simulink model "SyntheticDataSimulinkExample"  (R2017b)
settings: Solver=FixedStepDiscrete  StartTime=0.0  StopTime=14.34  FixedStep=0.1  RelTol=1e-3
undefined symbols (not defined in the file or in its folder): driving
libraries: drivinglib x12, drivingmisc x1
settings Model: Creator=The MathWorks, Inc.  LastModifiedBy=The MathWorks, Inc.
settings CodeAppCC: StateflowObjectComments=on

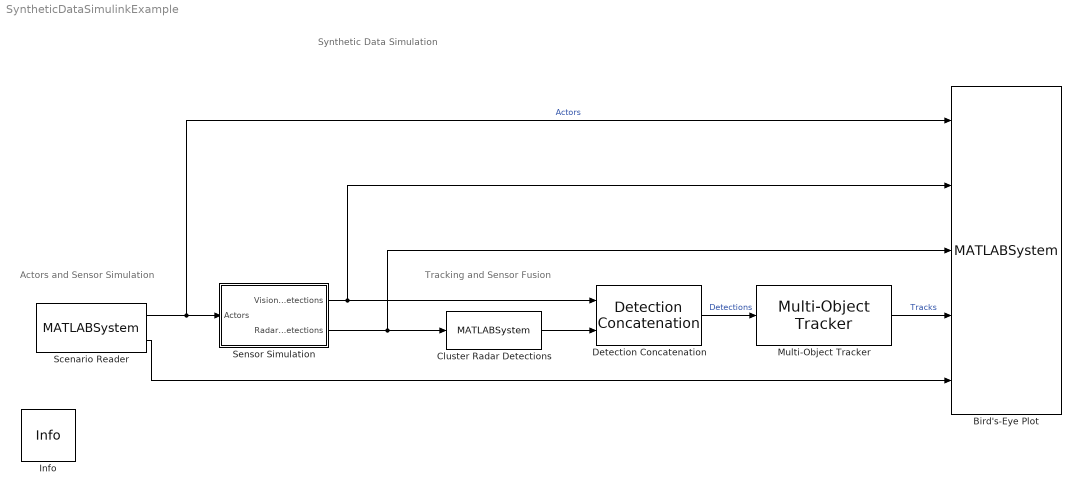
== system SyntheticDataSimulinkExample ==
  note: Tracking and Sensor Fusion
  note: Actors and Sensor Simulation
  note: Synthetic Data Simulation
  Bird's-Eye Plot : MATLABSystem  System=helperBirdsEyePlot  XLim=[ -60, 60 ]  YLim=[ -50, 50 ]  HasActors=on  HasVision=on  HasRadar=on  HasTracks=on  TrackPositionSelector=[ 1, 0, 0, 0, 0, 0; 0, 0, 1, 0, 0, 0 ]  TrackVelocitySelector=[ 0, 1, 0, 0, 0, 0; 0, 0, 0, 1, 0, 0 ]  HasMIO=off  HasRoads=on
      settings: ModelCloseFcn=helperCloseAll(gcb)
      mask Type: helperBirdsEyePlot
      mask Display:
      | disp(['Bird''s-Eye' char(10) 'Plot']);
      | port_label('input',1,'Actors');
      | port_label('input',2,'Vision');
      | port_label('input',3,'Radar');
      | port_label('input',4,'Tracks');
      | port_label('input',5,'Roads');
  Cluster Radar Detections : MATLABSystem  System=helperClusterDetections  ClusterSize=5  BusNameSource=Auto  SimulateUsing=Interpreted execution
      mask Type: helperClusterDetections
      mask Display:
      | disp(['Detection' char(10) 'Clustering']);
      | port_label('input',1,'In');
      | port_label('output',1,'Out');
  Detection Concatenation : drivinglib/Detection Concatenation  NumInputs=2  BusNameSource=Auto  BusName=BusDetectionConcatenation1  SimulateUsing=Interpreted execution
      settings: SourceProductName=Automated Driving System Toolbox
  Info : drivingmisc/Info  SystemSampleTime=-1
      settings: SourceProductName=Computer Vision System Toolbox  SourceProductBaseCode=VP
  Multi-Object Tracker : drivinglib/Multi-Object Tracker  FilterInitializationFcn=helperInitSimulinkDemoFilter  AssignmentThreshold=50  ConfirmationParameters=[ 2, 3 ]  NumCoastingUpdates=5  MaxNumTracks=20  MaxNumSensors=8  TimeInputSource=Auto  BusNameSource=Auto  BusName=BusMultiObjectTracker1  HasCostMatrixInput=off  TentativeTracksOutputPort=off  AllTracksOutputPort=off  SimulateUsing=Interpreted execution
      settings: SourceProductName=Automated Driving System Toolbox
  Scenario Reader : MATLABSystem  System=helperScenarioReader  ScenarioFileName=openLoopSimulinkScenario  EgoActorSource=Auto  EgoActorID=1  RoadBoundaries=on  BusNameSource=Auto  SimulateUsing=Interpreted execution
      mask Type: helperScenarioReader
      mask Display:
      | disp(['Scenario' char(10) 'Reader']);
      | port_label('output',1,'Actors');
      | port_label('output',2,'Roads');
  Sensor Simulation : Subsystem
  wires:
  Detection Concatenation/1 -> Multi-Object Tracker/1  "Detections"
  Scenario Reader/1 -> Bird's-Eye Plot/1, Sensor Simulation/1(Actors)  "Actors"
  Sensor Simulation/1(Vision Detections) -> Detection Concatenation/1, Bird's-Eye Plot/2
  Sensor Simulation/2(Radar Detections) -> Bird's-Eye Plot/3, Cluster Radar Detections/1
  Cluster Radar Detections/1 -> Detection Concatenation/2
  Scenario Reader/2 -> Bird's-Eye Plot/5
  Multi-Object Tracker/1 -> Bird's-Eye Plot/4  "Tracks"

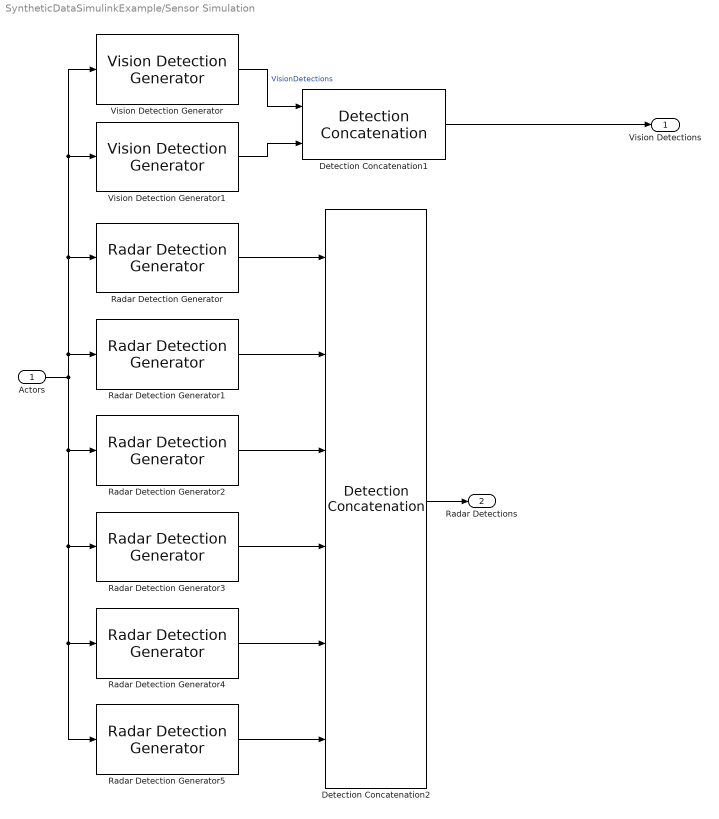
== system SyntheticDataSimulinkExample/Sensor Simulation ==
  Actors : Inport
  Detection Concatenation1 : drivinglib/Detection Concatenation  NumInputs=2  BusNameSource=Auto  BusName=BusDetectionConcatenation3  SimulateUsing=Interpreted execution
      settings: SourceProductName=Automated Driving System Toolbox
  Detection Concatenation2 : drivinglib/Detection Concatenation  NumInputs=6  BusNameSource=Auto  BusName=BusDetectionConcatenation2  SimulateUsing=Interpreted execution
      settings: SourceProductName=Automated Driving System Toolbox
  Radar Detection Generator : drivinglib/Radar Detection Generator  SensorIndex=3  UpdateInterval=0.1  SensorLocation=[ 3.7, 0 ]  Height=0.2  Yaw=0  Pitch=0  Roll=0  BusNameSource=Auto  BusName=BusRadarDetectionGenerator1  MaxNumDetectionsSource=Property  MaxNumDetections=50  DetectionCoordinates=Ego Cartesian  SimulateUsing=Interpreted execution  AzimuthResolution=4  ElevationResolution=10  RangeResolution=2.5  RangeRateResolution=0.5  AzimuthBiasFraction=0.1  ElevationBiasFraction=0.1  RangeBiasFraction=0.05  RangeRateBiasFraction=0.05  FieldOfView=[ 20, 5 ]  MaxRange=174  RangeRateLimits=[ -100, 100 ]  DetectionProbability=0.9  FalseAlarmRate=1e-6  ReferenceRange=100  ReferenceRCS=0  HasElevation=off  HasRangeRate=on  HasNoise=on  HasFalseAlarms=on  InitialSeedSource=Repeatable  InitialSeed=0  UsedSeed=driving.internal.SimulinkUtilities.seedManager(gcb)  ActorProfilesSource=Parameters  ActorProfilesParameters=driving.internal.ActorProfilesRadarParameters  ActorProfilesExpression=struct( 'ClassID', 0, 'Length', 4.7, 'Width', 1.8, 'Height', 1.4, 'OriginOffset', [ -1.35, 0, 0 ], 'RCSPattern', [ 10, 10; 10, 10 ], 'RCSAzimuthAngles', [ -180, 180 ], 'RCSElevationAngles', [ -90, 90 ] )
      settings: SourceProductName=Automated Driving System Toolbox
  Radar Detection Generator1 : drivinglib/Radar Detection Generator  SensorIndex=4  UpdateInterval=0.1  SensorLocation=[-1, 0 ]  Height=0.2  Yaw=180  Pitch=0  Roll=0  BusNameSource=Auto  BusName=BusRadarDetectionGenerator1  MaxNumDetectionsSource=Property  MaxNumDetections=50  DetectionCoordinates=Ego Cartesian  SimulateUsing=Interpreted execution  AzimuthResolution=4  ElevationResolution=10  RangeResolution=2.5  RangeRateResolution=0.5  AzimuthBiasFraction=0.1  ElevationBiasFraction=0.1  RangeBiasFraction=0.05  RangeRateBiasFraction=0.05  FieldOfView=[ 20, 5 ]  MaxRange=174  RangeRateLimits=[ -100, 100 ]  DetectionProbability=0.9  FalseAlarmRate=1e-6  ReferenceRange=100  ReferenceRCS=0  HasElevation=off  HasRangeRate=on  HasNoise=on  HasFalseAlarms=on  InitialSeedSource=Repeatable  InitialSeed=0  UsedSeed=driving.internal.SimulinkUtilities.seedManager(gcb)  ActorProfilesSource=Parameters  ActorProfilesParameters=driving.internal.ActorProfilesRadarParameters  ActorProfilesExpression=struct( 'ClassID', 0, 'Length', 4.7, 'Width', 1.8, 'Height', 1.4, 'OriginOffset', [ -1.35, 0, 0 ], 'RCSPattern', [ 10, 10; 10, 10 ], 'RCSAzimuthAngles', [ -180, 180 ], 'RCSElevationAngles', [ -90, 90 ] )
      settings: SourceProductName=Automated Driving System Toolbox
  Radar Detection Generator2 : drivinglib/Radar Detection Generator  SensorIndex=5  UpdateInterval=0.1  SensorLocation=[0, 0.90 ]  Height=0.2  Yaw=120  Pitch=0  Roll=0  BusNameSource=Auto  BusName=BusRadarDetectionGenerator1  MaxNumDetectionsSource=Property  MaxNumDetections=50  DetectionCoordinates=Ego Cartesian  SimulateUsing=Interpreted execution  AzimuthResolution=4  ElevationResolution=10  RangeResolution=2.5  RangeRateResolution=0.5  AzimuthBiasFraction=0.1  ElevationBiasFraction=0.1  RangeBiasFraction=0.05  RangeRateBiasFraction=0.05  FieldOfView=[ 90, 5 ]  MaxRange=30  RangeRateLimits=[ -100, 100 ]  DetectionProbability=0.9  FalseAlarmRate=1e-6  ReferenceRange=100  ReferenceRCS=0  HasElevation=off  HasRangeRate=on  HasNoise=on  HasFalseAlarms=on  InitialSeedSource=Repeatable  InitialSeed=0  UsedSeed=driving.internal.SimulinkUtilities.seedManager(gcb)  ActorProfilesSource=Parameters  ActorProfilesParameters=driving.internal.ActorProfilesRadarParameters  ActorProfilesExpression=struct( 'ClassID', 0, 'Length', 4.7, 'Width', 1.8, 'Height', 1.4, 'OriginOffset', [ -1.35, 0, 0 ], 'RCSPattern', [ 10, 10; 10, 10 ], 'RCSAzimuthAngles', [ -180, 180 ], 'RCSElevationAngles', [ -90, 90 ] )
      settings: SourceProductName=Automated Driving System Toolbox
  Radar Detection Generator3 : drivinglib/Radar Detection Generator  SensorIndex=6  UpdateInterval=0.1  SensorLocation=[ 0, -0.90 ]  Height=0.2  Yaw=-120  Pitch=0  Roll=0  BusNameSource=Auto  BusName=BusRadarDetectionGenerator1  MaxNumDetectionsSource=Property  MaxNumDetections=50  DetectionCoordinates=Ego Cartesian  SimulateUsing=Interpreted execution  AzimuthResolution=4  ElevationResolution=10  RangeResolution=2.5  RangeRateResolution=0.5  AzimuthBiasFraction=0.1  ElevationBiasFraction=0.1  RangeBiasFraction=0.05  RangeRateBiasFraction=0.05  FieldOfView=[ 90, 5 ]  MaxRange=30  RangeRateLimits=[ -100, 100 ]  DetectionProbability=0.9  FalseAlarmRate=1e-6  ReferenceRange=100  ReferenceRCS=0  HasElevation=off  HasRangeRate=on  HasNoise=on  HasFalseAlarms=on  InitialSeedSource=Repeatable  InitialSeed=0  UsedSeed=driving.internal.SimulinkUtilities.seedManager(gcb)  ActorProfilesSource=Parameters  ActorProfilesParameters=driving.internal.ActorProfilesRadarParameters  ActorProfilesExpression=struct( 'ClassID', 0, 'Length', 4.7, 'Width', 1.8, 'Height', 1.4, 'OriginOffset', [ -1.35, 0, 0 ], 'RCSPattern', [ 10, 10; 10, 10 ], 'RCSAzimuthAngles', [ -180, 180 ], 'RCSElevationAngles', [ -90, 90 ] )
      settings: SourceProductName=Automated Driving System Toolbox
  Radar Detection Generator4 : drivinglib/Radar Detection Generator  SensorIndex=7  UpdateInterval=0.1  SensorLocation=[2.8, 0.9 ]  Height=0.2  Yaw=60  Pitch=0  Roll=0  BusNameSource=Auto  BusName=BusRadarDetectionGenerator1  MaxNumDetectionsSource=Property  MaxNumDetections=50  DetectionCoordinates=Ego Cartesian  SimulateUsing=Interpreted execution  AzimuthResolution=4  ElevationResolution=10  RangeResolution=2.5  RangeRateResolution=0.5  AzimuthBiasFraction=0.1  ElevationBiasFraction=0.1  RangeBiasFraction=0.05  RangeRateBiasFraction=0.05  FieldOfView=[ 90, 5 ]  MaxRange=30  RangeRateLimits=[ -100, 100 ]  DetectionProbability=0.9  FalseAlarmRate=1e-6  ReferenceRange=100  ReferenceRCS=0  HasElevation=off  HasRangeRate=on  HasNoise=on  HasFalseAlarms=on  InitialSeedSource=Repeatable  InitialSeed=0  UsedSeed=driving.internal.SimulinkUtilities.seedManager(gcb)  ActorProfilesSource=Parameters  ActorProfilesParameters=driving.internal.ActorProfilesRadarParameters  ActorProfilesExpression=struct( 'ClassID', 0, 'Length', 4.7, 'Width', 1.8, 'Height', 1.4, 'OriginOffset', [ -1.35, 0, 0 ], 'RCSPattern', [ 10, 10; 10, 10 ], 'RCSAzimuthAngles', [ -180, 180 ], 'RCSElevationAngles', [ -90, 90 ] )
      settings: SourceProductName=Automated Driving System Toolbox
  Radar Detection Generator5 : drivinglib/Radar Detection Generator  SensorIndex=8  UpdateInterval=0.1  SensorLocation=[ 2.8, -0.9 ]  Height=0.2  Yaw=-60  Pitch=0  Roll=0  BusNameSource=Auto  BusName=BusRadarDetectionGenerator1  MaxNumDetectionsSource=Property  MaxNumDetections=50  DetectionCoordinates=Ego Cartesian  SimulateUsing=Interpreted execution  AzimuthResolution=4  ElevationResolution=10  RangeResolution=2.5  RangeRateResolution=0.5  AzimuthBiasFraction=0.1  ElevationBiasFraction=0.1  RangeBiasFraction=0.05  RangeRateBiasFraction=0.05  FieldOfView=[ 90, 5 ]  MaxRange=30  RangeRateLimits=[ -100, 100 ]  DetectionProbability=0.9  FalseAlarmRate=1e-6  ReferenceRange=100  ReferenceRCS=0  HasElevation=off  HasRangeRate=on  HasNoise=on  HasFalseAlarms=on  InitialSeedSource=Repeatable  InitialSeed=0  UsedSeed=driving.internal.SimulinkUtilities.seedManager(gcb)  ActorProfilesSource=Parameters  ActorProfilesParameters=driving.internal.ActorProfilesRadarParameters  ActorProfilesExpression=struct( 'ClassID', 0, 'Length', 4.7, 'Width', 1.8, 'Height', 1.4, 'OriginOffset', [ -1.35, 0, 0 ], 'RCSPattern', [ 10, 10; 10, 10 ], 'RCSAzimuthAngles', [ -180, 180 ], 'RCSElevationAngles', [ -90, 90 ] )
      settings: SourceProductName=Automated Driving System Toolbox
  Vision Detection Generator : drivinglib/Vision Detection Generator  SensorIndex=1  UpdateInterval=0.1  SensorLocation=[ 2.1, 0 ]  Height=1.1  Yaw=0  Pitch=1  Roll=0  BusNameSource=Auto  BusName=BusVisionDetectionGenerator1  MaxNumDetectionsSource=Property  MaxNumDetections=20  DetectionCoordinates=Ego Cartesian  SimulateUsing=Interpreted execution  BoundingBoxAccuracy=5  ProcessNoiseIntensity=5  HasNoise=on  MaxRange=150  MaxSpeed=50  MaxAllowedOcclusion=0.5  MinObjectImageSize=[ 15, 15 ]  DetectionProbability=0.9  FalsePositivesPerImage=0.1  InitialSeedSource=Repeatable  InitialSeed=0  UsedSeed=driving.internal.SimulinkUtilities.seedManager(gcb)  ActorProfilesSource=Parameters  ActorProfilesParameters=driving.internal.ActorProfilesParameters  ActorProfilesExpression=struct( 'ClassID', 0, 'Length', 4.7, 'Width', 1.8, 'Height', 1.4, 'OriginOffset', [ -1.35, 0, 0 ] )  Intrinsics=driving.internal.cameraIntrinsics
      settings: SourceProductName=Automated Driving System Toolbox
  Vision Detection Generator1 : drivinglib/Vision Detection Generator  SensorIndex=2  UpdateInterval=0.1  SensorLocation=[ 0.56, 0 ]  Height=1.1  Yaw=180  Pitch=1  Roll=0  BusNameSource=Auto  BusName=BusVisionDetectionGenerator1  MaxNumDetectionsSource=Property  MaxNumDetections=20  DetectionCoordinates=Ego Cartesian  SimulateUsing=Interpreted execution  BoundingBoxAccuracy=5  ProcessNoiseIntensity=5  HasNoise=on  MaxRange=150  MaxSpeed=50  MaxAllowedOcclusion=0.5  MinObjectImageSize=[ 15, 15 ]  DetectionProbability=0.9  FalsePositivesPerImage=0.1  InitialSeedSource=Repeatable  InitialSeed=0  UsedSeed=driving.internal.SimulinkUtilities.seedManager(gcb)  ActorProfilesSource=Parameters  ActorProfilesParameters=driving.internal.ActorProfilesParameters  ActorProfilesExpression=struct( 'ClassID', 0, 'Length', 4.7, 'Width', 1.8, 'Height', 1.4, 'OriginOffset', [ -1.35, 0, 0 ] )  Intrinsics=driving.internal.cameraIntrinsics
      settings: SourceProductName=Automated Driving System Toolbox
  Vision Detections : Outport
  Radar Detections : Outport  Port=2
  wires:
  Vision Detection Generator/1 -> Detection Concatenation1/1  "VisionDetections"
  Radar Detection Generator3/1 -> Detection Concatenation2/4
  Detection Concatenation1/1 -> Vision Detections/1
  Radar Detection Generator4/1 -> Detection Concatenation2/5
  Detection Concatenation2/1 -> Radar Detections/1
  Radar Detection Generator1/1 -> Detection Concatenation2/2
  Radar Detection Generator5/1 -> Detection Concatenation2/6
  Radar Detection Generator/1 -> Detection Concatenation2/1
  Radar Detection Generator2/1 -> Detection Concatenation2/3
  Vision Detection Generator1/1 -> Detection Concatenation1/2
  Actors/1 -> Vision Detection Generator/1, Vision Detection Generator1/1, Radar Detection Generator/1, Radar Detection Generator1/1, Radar Detection Generator5/1, Radar Detection Generator4/1, Radar Detection Generator3/1, Radar Detection Generator2/1
